simulink model "a22_sim"  (R2014a)
settings: Solver=ode45  StartTime=0.0  StopTime=10.0  RelTol=1e-3
values from neighbouring files (symbols this model uses):
  C = 1e-6    (= 1e-06)    [a08.m]    (also in a22.m = 0.01)
  R = 1e3    (= 1000)    [a08.m]    (also in a22.m)
settings Model: Creator=s65556  LastModifiedBy=s65556

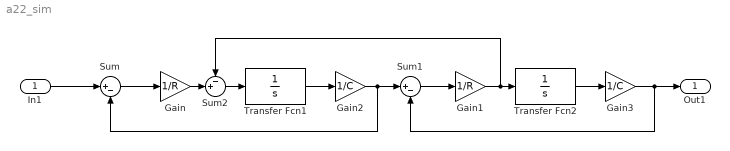
== system a22_sim ==
  In1 : Inport
  Gain : Gain  Gain=1/R
  Gain1 : Gain  Gain=1/R
  Gain2 : Gain  Gain=1/C
  Gain3 : Gain  Gain=1/C
  Sum : Sum  Inputs=|+-
  Sum1 : Sum  Inputs=|+-
  Sum2 : Sum  Inputs=-+|
  Transfer Fcn1 : TransferFcn  Denominator=[1 0]
  Transfer Fcn2 : TransferFcn  Denominator=[1 0]
  Out1 : Outport
  wires:
  In1/1 -> Sum/1
  Sum/1 -> Gain/1
  Transfer Fcn1/1 -> Gain2/1
  Gain2/1 -> Sum/2, Sum1/1
  Sum1/1 -> Gain1/1
  Gain1/1 -> Sum2/1, Transfer Fcn2/1
  Transfer Fcn2/1 -> Gain3/1
  Gain3/1 -> Sum1/2, Out1/1
  Gain/1 -> Sum2/2
  Sum2/1 -> Transfer Fcn1/1
